simulink model "LQG_Observer"  (R2020a)
settings: Solver=VariableStepAuto  StartTime=0.0  StopTime=10.0  RelTol=1e-3
values from neighbouring files (symbols this model uses):
  A = [0, 1; 4.1*10^4, 0]    [LQG_Observer_params.m]    (also in kalman_observer_params.m)
  B = [0; -9.12]    [LQG_Observer_params.m]    (also in kalman_observer_params.m)
  C = [1 0;0 1]    [LQG_Observer_params.m]    (also in kalman_observer_params.m)
  K_u = inv(R)*B'*P    [kalman_observer_params.m]
  L = place(A',C', eig_Kc)    [LQG_Observer_params.m]    (also in kalman_observer_params.m = K_k)
settings Model: Creator=prans  LastModifiedBy=prans

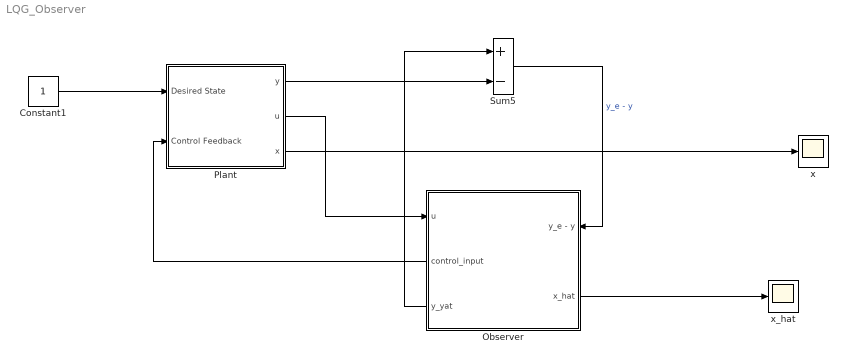
== system LQG_Observer ==
  Constant1 : Constant
  Observer : Subsystem
      settings: PortSchema="{\"entries\":[{\"content\":{\"sides\":[{\"content\":{\"connectorIds\":[\"In1\",\"Out2\",\"Out3\"]},\"type\":\"ConnectorPlacement.EquallySpacedRectSide\",\"uuid\":\"a9f7231f-0ea7-4ecf-9f4d-3b1190901673\"},{\"content\":{\"connectorIds\":[\"In2\",\"Out1\"],\"side\":\"RIGHT\"},\"type\":\"ConnectorPlacement.EquallySpacedRectSide\",\"uuid\":\"d8eefaaa-fd2b-41d2-a0dc-5def7f7cb866\"},{\"content\":{\"connectorIds\":[],\"side\":\"TOP\"},\"type\":\"ConnectorPlacement.EquallySpacedRectSide\",\"uuid\":\"31c1f2f2-3408-4380-abb9-8d04f7653d19\"}]},\"type\":\"ConnectorPlacement.EquallySpacedConnector\",\"uuid\":\"c5ec393a-74ff-441f-a8d4-81f60b397274\"}],\"packageUris\":[\"http://schema.mathworks.com/mf0/Connector/19700101\"],\"version\":\"1.0\"}"
  Plant : Subsystem
  Sum5 : Sum  Inputs=+-
  x : Scope
  x_hat : Scope
  wires:
  Constant1/1 -> Plant/1(Desired State)
  Plant/1(y) -> Sum5/2
  Sum5/1 -> Observer/2(y_e - y)  "y_e - y"
  Plant/2(u) -> Observer/1(u)
  Observer/2(control_input) -> Plant/2(Control Feedback)
  Observer/3(y_yat) -> Sum5/1
  Observer/1(x_hat) -> x_hat/1
  Plant/3(x) -> x/1

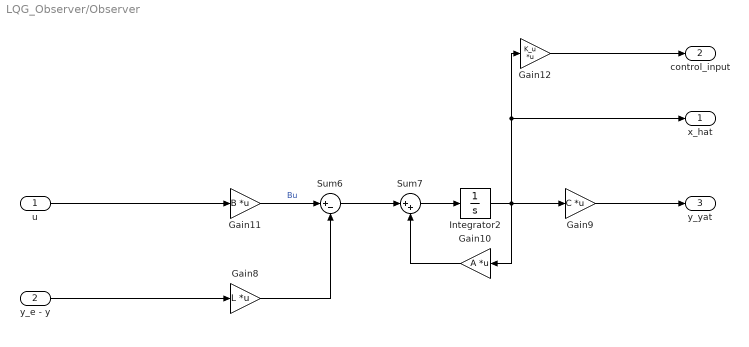
== system LQG_Observer/Observer ==
  u : Inport
  y_e - y : Inport  Port=2
  Gain10 : Gain  Gain=A  Multiplication=Matrix(K*u)
  Gain11 : Gain  Gain=B  Multiplication=Matrix(K*u)
  Gain12 : Gain  Gain=K_u  Multiplication=Matrix(K*u)
  Gain8 : Gain  Gain=L  Multiplication=Matrix(K*u)
  Gain9 : Gain  Gain=C  Multiplication=Matrix(K*u)
  Integrator2 : Integrator
  Sum6 : Sum  Inputs=|+-
  Sum7 : Sum  Inputs=|++
  x_hat : Outport
  control_input : Outport  Port=2
  y_yat : Outport  Port=3
  wires:
  Integrator2/1 -> Gain9/1, x_hat/1, Gain12/1, Gain10/1
  Gain8/1 -> Sum6/2
  Sum6/1 -> Sum7/1
  Gain11/1 -> Sum6/1  "Bu"
  Gain10/1 -> Sum7/2
  Sum7/1 -> Integrator2/1
  y_e - y/1 -> Gain8/1
  Gain12/1 -> control_input/1
  u/1 -> Gain11/1
  Gain9/1 -> y_yat/1

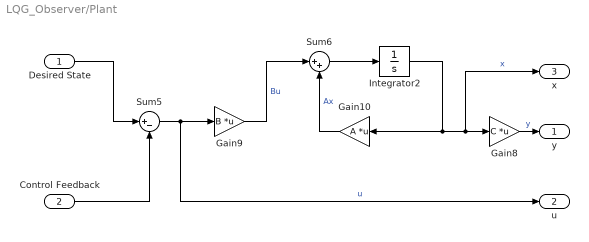
== system LQG_Observer/Plant ==
  Desired State : Inport
  Control Feedback : Inport  Port=2
  Gain10 : Gain  Gain=A  Multiplication=Matrix(K*u)
  Gain8 : Gain  Gain=C  Multiplication=Matrix(K*u)
  Gain9 : Gain  Gain=B  Multiplication=Matrix(K*u)
  Integrator2 : Integrator
  Sum5 : Sum  Inputs=|+-
  Sum6 : Sum  Inputs=|++
  y : Outport
  u : Outport  Port=2
  x : Outport  Port=3
  wires:
  Integrator2/1 -> Gain10/1, x/1, Gain8/1  "x"
  Sum6/1 -> Integrator2/1
  Gain8/1 -> y/1  "y"
  Desired State/1 -> Sum5/1
  Gain9/1 -> Sum6/1  "Bu"
  Gain10/1 -> Sum6/2  "Ax"
  Sum5/1 -> u/1, Gain9/1  "u"
  Control Feedback/1 -> Sum5/2
